simulink model "MRAC_generalizado2"  (Simulink 10.3)
settings: Solver=ode45  StartTime=10  StopTime=20  RelTol=1e-3  AbsTol=1e-6
values from neighbouring files (symbols this model uses):
  Af = zeros(n-1,n-1)    [MRAC_generalizado.m]    (also in MRAC_generalizado_nstar_1.m = zeros(nf); Af(1:nf-1, 2:nf) = eye(nf-1); Af(end, :) = -flipl; MRAC_generalizado_nstar_2.m = zeros(nf); Af(1:nf-1, 2:nf) = eye(nf-1); Af(end, :) = -flipl)
  Aq = 2    [MRAC_generalizado_nstar_1.m]    (also in MRAC_generalizado_nstar_2.m = 5)
  As = 5    [MRAC_generalizado_nstar_1.m]    (also in MRAC_generalizado_nstar_2.m = 3)
  Bf = zeros(n-1,1)    [MRAC_generalizado.m]    (also in MRAC_generalizado_nstar_1.m = zeros(nf,1); Bf(end) = 1; MRAC_generalizado_nstar_2.m = zeros(nf,1); Bf(end) = 1)
  DC = 2    [MRAC_generalizado_nstar_1.m]    (also in MRAC_generalizado_nstar_2.m)
  gamma = 10*eye(2*n)    [MRAC_generalizado_nstar_1.m]    (also in MRAC_generalizado_nstar_2.m)
  kp = 2    [MRAC_generalizado.m]    (also in MRAC_generalizado_nstar_1.m = 2 + rand(); MRAC_generalizado_nstar_2.m; controle2DOF.m = N_p(find(N_p ~= 0, 1, 'first')); controle2DOF_nstar2.m = N_p(find(N_p ~= 0, 1, 'first')))
  l0 = -zeros_L    (= 2)    [MRAC_generalizado_nstar_2.m]
  st = 0.01    [MRAC_generalizado_nstar_1.m]    (also in MRAC_generalizado_nstar_2.m)
  theta0 = 0.95*theta_star    [MRAC_generalizado_nstar_1.m]    (also in MRAC_generalizado_nstar_2.m)
  wq = 0.1*pi    (= 0.314159265359)    [MRAC_generalizado_nstar_1.m]    (also in MRAC_generalizado_nstar_2.m)
  ws = 1    [MRAC_generalizado_nstar_1.m]    (also in MRAC_generalizado_nstar_2.m = 0.628318530718)
libraries: cstblocks x2
settings Model: LogicAnalyzerSignalOrdering=7416a645-b114-49ae-ab40-1077c7b9da29,10dc0d5a-646b-48fc-bc01-8c278f0b01d3,0804b0ab-6626-4093-842a-42967a9eb430  Creator=Ramon  LastModifiedBy=linco  MultithreadedSim=on
settings SolverCC: AutoScaleAbsTol=off
settings DataIOCC: SaveOutput=off  SaveTime=off
settings OptimizationCC: BlockReduction=off  BooleanDataType=off  InitFltsAndDblsToZero=on
settings DebuggingCC: SaveWithParameterizedLinksMsg=none  SignalResolutionControl=TryResolveAllWithWarning  MultiTaskDSMMsg=warning  MultiTaskCondExecSysMsg=none
settings HardwareCC: TargetUnknown=on
settings RTWCC: TemplateMakefile=grt_vc.tmf

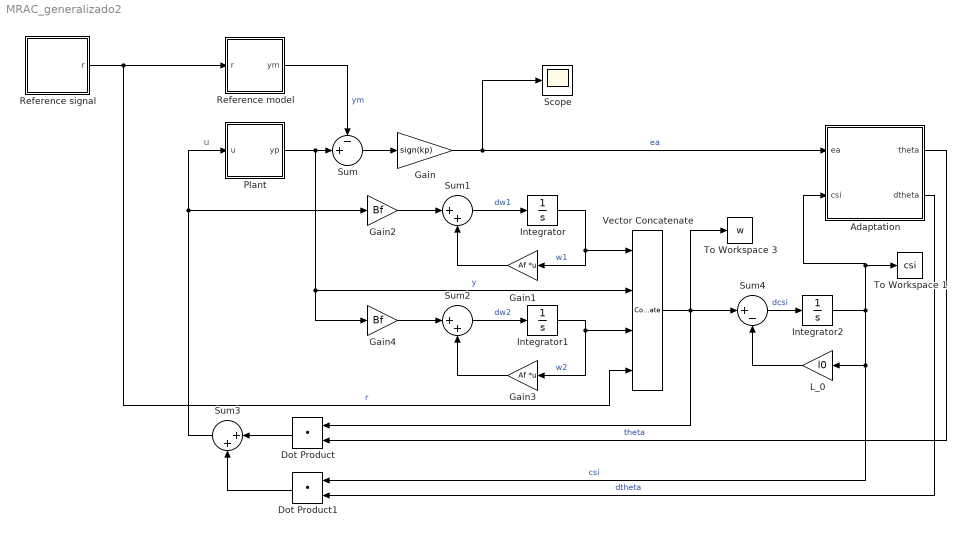
== system MRAC_generalizado2 ==
  note: u
  Adaptation : Subsystem
  Dot Product : DotProduct  InputSameDT=on  OutDataTypeStr=Inherit: Inherit via internal rule
  Dot Product1 : DotProduct  InputSameDT=on  OutDataTypeStr=Inherit: Inherit via internal rule
  Gain : Gain  Gain=sign(kp)
  Gain1 : Gain  Gain=Af  Multiplication=Matrix(K*u) (u vector)
  Gain2 : Gain  Gain=Bf
  Gain3 : Gain  Gain=Af  Multiplication=Matrix(K*u) (u vector)
  Gain4 : Gain  Gain=Bf
  Integrator : Integrator
  Integrator1 : Integrator
  Integrator2 : Integrator
  L_0 : Gain  Gain=l0
  Plant : Subsystem
  Reference model : Subsystem
  Reference signal : Subsystem
  Scope : Scope
  Sum : Sum  Inputs=-+|  InputSameDT=on  SaturateOnIntegerOverflow=on  OutDataTypeStr=Inherit: Same as first input
  Sum1 : Sum  Inputs=|++  InputSameDT=on  SaturateOnIntegerOverflow=on  OutDataTypeStr=Inherit: Same as first input
  Sum2 : Sum  Inputs=|++  InputSameDT=on  SaturateOnIntegerOverflow=on  OutDataTypeStr=Inherit: Same as first input
  Sum3 : Sum  Inputs=|++  InputSameDT=on  SaturateOnIntegerOverflow=on  OutDataTypeStr=Inherit: Same as first input
  Sum4 : Sum  Inputs=|+-  InputSameDT=on  SaturateOnIntegerOverflow=on  OutDataTypeStr=Inherit: Same as first input
  To Workspace 1 : ToWorkspace  VariableName=csi  SampleTime=st
  To Workspace 3 : ToWorkspace  VariableName=w  SampleTime=st
  Vector Concatenate : Concatenate  NumInputs=4
  wires:
  Reference model/1(ym) -> Sum/1  "ym"
  Plant/1(yp) -> Gain4/1, Vector Concatenate/2, Sum/2  "y"
  Sum3/1 -> Plant/1(u), Gain2/1
  Adaptation/1(theta) -> Dot Product/2  "theta"
  Gain/1 -> Scope/1, Adaptation/1(ea)  "ea"
  Sum/1 -> Gain/1
  Sum1/1 -> Integrator/1  "dw1"
  Gain2/1 -> Sum1/1
  Integrator/1 -> Vector Concatenate/1, Gain1/1  "w1"
  Gain1/1 -> Sum1/2
  Sum2/1 -> Integrator1/1  "dw2"
  Reference signal/1(r) -> Vector Concatenate/4, Reference model/1(r)  "r"
  Integrator1/1 -> Gain3/1, Vector Concatenate/3  "w2"
  Gain3/1 -> Sum2/2
  Gain4/1 -> Sum2/1
  Vector Concatenate/1 -> To Workspace 3/1, Sum4/1, Dot Product/1
  Integrator2/1 -> To Workspace 1/1, Adaptation/2(csi), Dot Product1/1, L_0/1  "csi"
  Sum4/1 -> Integrator2/1  "dcsi"
  L_0/1 -> Sum4/2
  Dot Product/1 -> Sum3/1
  Dot Product1/1 -> Sum3/2
  Adaptation/2(dtheta) -> Dot Product1/2  "dtheta"

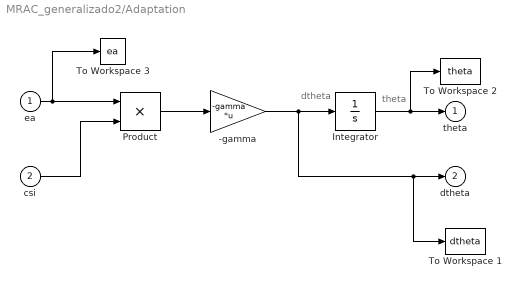
== system MRAC_generalizado2/Adaptation ==
  note: theta
  note: dtheta
  ea : Inport  PortDimensions=1
  csi : Inport  Port=2
  -gamma : Gain  Gain=-gamma  Multiplication=Matrix(K*u) (u vector)  SaturateOnIntegerOverflow=on  OutDataTypeStr=Inherit: Same as input  ParamDataTypeStr=Inherit: Same as input
  Integrator : Integrator  InitialCondition=theta0
  Product : Product  InputSameDT=on  RndMeth=Zero  SaturateOnIntegerOverflow=on  OutDataTypeStr=Inherit: Same as first input
  To Workspace 1 : ToWorkspace  VariableName=dtheta  SampleTime=st
  To Workspace 2 : ToWorkspace  VariableName=theta  SampleTime=st
  To Workspace 3 : ToWorkspace  VariableName=ea  SampleTime=st
  theta : Outport  InitialOutput=0  VectorParamsAs1DForOutWhenUnconnected=off
  dtheta : Outport  Port=2  InitialOutput=0  VectorParamsAs1DForOutWhenUnconnected=off
  wires:
  Integrator/1 -> To Workspace 2/1, theta/1
  -gamma/1 -> To Workspace 1/1, dtheta/1, Integrator/1
  ea/1 -> Product/1, To Workspace 3/1
  Product/1 -> -gamma/1
  csi/1 -> Product/2

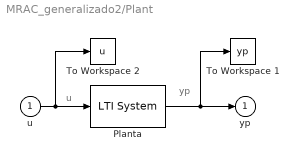
== system MRAC_generalizado2/Plant ==
  note: yp
  note: u
  u : Inport
  Planta : cstblocks/LTI System  sys=P  IC=x0
  To Workspace 1 : ToWorkspace  VariableName=yp  SampleTime=st
  To Workspace 2 : ToWorkspace  VariableName=u  SampleTime=st
  yp : Outport  InitialOutput=0  VectorParamsAs1DForOutWhenUnconnected=off
  wires:
  u/1 -> To Workspace 2/1, Planta/1
  Planta/1 -> yp/1, To Workspace 1/1

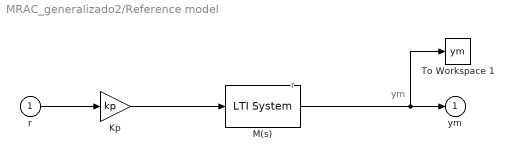
== system MRAC_generalizado2/Reference model ==
  note: r
  note: ym
  r : Inport
  Kp : Gain  Gain=kp
  M(s) : cstblocks/LTI System  sys=M  IC=xm0
  To Workspace 1 : ToWorkspace  VariableName=ym  SampleTime=st
  ym : Outport  InitialOutput=0  VectorParamsAs1DForOutWhenUnconnected=off
  wires:
  M(s)/1 -> To Workspace 1/1, ym/1
  Kp/1 -> M(s)/1
  r/1 -> Kp/1

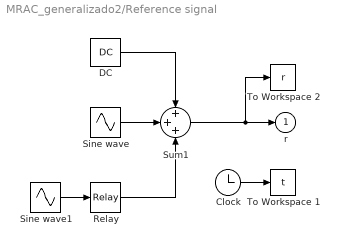
== system MRAC_generalizado2/Reference signal ==
  Clock : Clock
  DC : Constant  Value=DC
  Relay : Relay  OnOutputValue=Aq  OffOutputValue=-Aq
  Sine wave : Sin  Amplitude=As  Frequency=ws  SampleTime=0
  Sine wave1 : Sin  Frequency=wq  SampleTime=0
  Sum1 : Sum  Inputs=+++  InputSameDT=on  SaturateOnIntegerOverflow=on  OutDataTypeStr=Inherit: Same as first input
  To Workspace 1 : ToWorkspace  VariableName=t  SampleTime=st
  To Workspace 2 : ToWorkspace  VariableName=r  SampleTime=st
  r : Outport  InitialOutput=0  VectorParamsAs1DForOutWhenUnconnected=off
  wires:
  DC/1 -> Sum1/1
  Sum1/1 -> r/1, To Workspace 2/1
  Clock/1 -> To Workspace 1/1
  Sine wave/1 -> Sum1/2
  Relay/1 -> Sum1/3
  Sine wave1/1 -> Relay/1
